simulink model "DvrSimKeybdGD_cs_old"  (R2016a)
settings: Solver=ode5  SolverMode=SingleTasking  StartTime=0.0  StopTime=inf  FixedStep=1/1000  RelTol=1e-3
PreLoadFcn:
  | mbxruntime.callbacks.PreLoadFcn(bdroot);
PostLoadFcn:
  | mbxruntime.callbacks.PostLoadFcn(bdroot);
InitFcn:
  | mbxruntime.callbacks.InitFcn(bdroot);
StartFcn:
  | mbxruntime.callbacks.StartFcn(bdroot);
StopFcn:
  | mbxruntime.callbacks.StopFcn(bdroot);
model workspace (MAT data in the model file):
  mbox_table : struct (value not decoded)
  model_closed = 0
  sim_status = 0
undefined symbols (not defined in the file or in its folder): BMotor1, BMotor2, BrkDelayTime, DControlB, Delay1, Delay2, DiscIntNeverNeededParam, IControlB, JMotor1, JMotor2, PControlB, PreScanCarSimLoadFcn, ratioGearF, ratioGearR, TorqDelayTime, Tstep
undefined symbols (not defined in the file): SteeringColumn, SteeringWheel, WheelL0, WheelL1, WheelR0, WheelR1
libraries: PreScanSimulinkLibrary x35, simulink_extras x26, simulink x26, MyLib x3, Solver_SF x2, pil_lib x1, PreScanUsefulBlocks x1
(part 5 of 12)

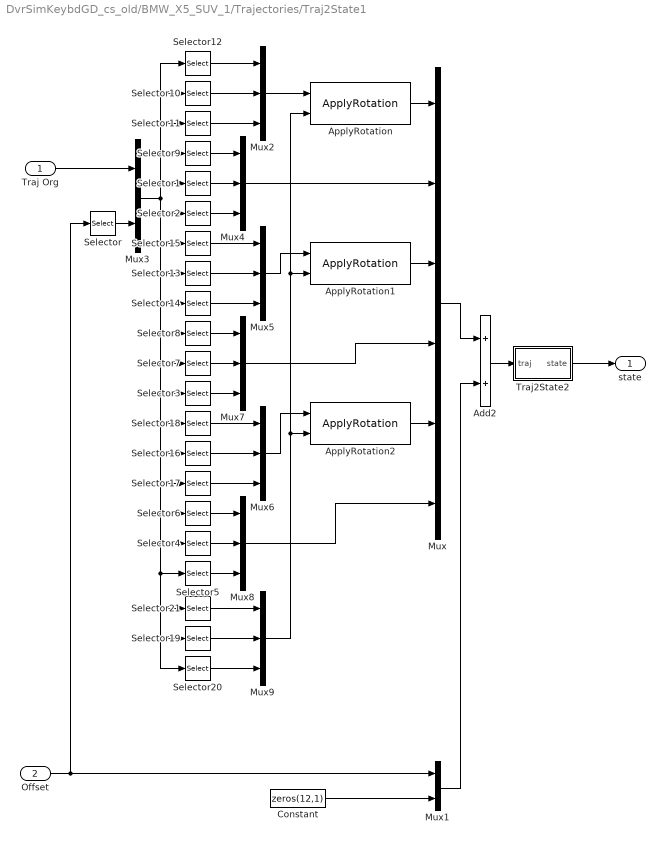
== system DvrSimKeybdGD_cs_old/BMW_X5_SUV_1/Trajectories/Traj2State1 ==
  Traj Org : Inport
  Offset : Inport  Port=2
  Add2 : Sum
  ApplyRotation : PreScanSimulinkLibrary/ApplyRotation
  ApplyRotation1 : PreScanSimulinkLibrary/ApplyRotation
  ApplyRotation2 : PreScanSimulinkLibrary/ApplyRotation
  Constant : Constant  Value=zeros(12,1)
  Mux : Mux  Inputs=6
  Mux1 : Mux  Inputs=2
  Mux{2,4..9} (7 alike) : Mux  Inputs=3
  Mux3 : Mux  Inputs=2
  Selector : Selector  InputPortWidth=6  IndexOptions=Index vector (dialog)  Indices=[4 5 6]  OutputSizes=1
  Selector1 : Selector  InputPortWidth=21  IndexOptions=Index vector (dialog)  Indices=[5]  OutputSizes=1
  Selector10 : Selector  InputPortWidth=21  IndexOptions=Index vector (dialog)  Indices=[2]  OutputSizes=1
  Selector11 : Selector  InputPortWidth=21  IndexOptions=Index vector (dialog)  Indices=[3]  OutputSizes=1
  Selector12 : Selector  InputPortWidth=21  IndexOptions=Index vector (dialog)  Indices=[1]  OutputSizes=1
  Selector13 : Selector  InputPortWidth=21  IndexOptions=Index vector (dialog)  Indices=[8]  OutputSizes=1
  Selector14 : Selector  InputPortWidth=21  IndexOptions=Index vector (dialog)  Indices=[9]  OutputSizes=1
  Selector15 : Selector  InputPortWidth=21  IndexOptions=Index vector (dialog)  Indices=[7]  OutputSizes=1
  Selector16 : Selector  InputPortWidth=21  IndexOptions=Index vector (dialog)  Indices=[14]  OutputSizes=1
  Selector17 : Selector  InputPortWidth=21  IndexOptions=Index vector (dialog)  Indices=[15]  OutputSizes=1
  Selector18 : Selector  InputPortWidth=21  IndexOptions=Index vector (dialog)  Indices=[13]  OutputSizes=1
  Selector19 : Selector  InputPortWidth=21  IndexOptions=Index vector (dialog)  Indices=[20]  OutputSizes=1
  Selector2 : Selector  InputPortWidth=21  IndexOptions=Index vector (dialog)  Indices=[6]  OutputSizes=1
  Selector20 : Selector  InputPortWidth=21  IndexOptions=Index vector (dialog)  Indices=[21]  OutputSizes=1
  Selector21 : Selector  InputPortWidth=21  IndexOptions=Index vector (dialog)  Indices=[19]  OutputSizes=1
  Selector3 : Selector  InputPortWidth=21  IndexOptions=Index vector (dialog)  Indices=[12]  OutputSizes=1
  Selector4 : Selector  InputPortWidth=21  IndexOptions=Index vector (dialog)  Indices=[17]  OutputSizes=1
  Selector5 : Selector  InputPortWidth=21  IndexOptions=Index vector (dialog)  Indices=[18]  OutputSizes=1
  Selector6 : Selector  InputPortWidth=21  IndexOptions=Index vector (dialog)  Indices=[16]  OutputSizes=1
  Selector7 : Selector  InputPortWidth=21  IndexOptions=Index vector (dialog)  Indices=[11]  OutputSizes=1
  Selector8 : Selector  InputPortWidth=21  IndexOptions=Index vector (dialog)  Indices=[10]  OutputSizes=1
  Selector9 : Selector  InputPortWidth=21  IndexOptions=Index vector (dialog)  Indices=[4]  OutputSizes=1
  Traj2State2 : Subsystem
  state : Outport
  wires:
  Mux9/1 -> ApplyRotation2/2, ApplyRotation1/2, ApplyRotation/2
  Selector20/1 -> Mux9/3
  Selector19/1 -> Mux9/2
  Selector21/1 -> Mux9/1
  Selector5/1 -> Mux8/3
  Selector4/1 -> Mux8/2
  Selector6/1 -> Mux8/1
  Mux8/1 -> Mux/6
  Mux6/1 -> ApplyRotation2/1
  Mux7/1 -> Mux/4
  ApplyRotation2/1 -> Mux/5
  Selector3/1 -> Mux7/3
  Selector7/1 -> Mux7/2
  Selector8/1 -> Mux7/1
  Mux4/1 -> Mux/2
  Mux5/1 -> ApplyRotation1/1
  ApplyRotation1/1 -> Mux/3
  Mux2/1 -> ApplyRotation/1
  ApplyRotation/1 -> Mux/1
  Selector2/1 -> Mux4/3
  Selector1/1 -> Mux4/2
  Selector9/1 -> Mux4/1
  Selector17/1 -> Mux6/3
  Selector16/1 -> Mux6/2
  Selector18/1 -> Mux6/1
  Selector14/1 -> Mux5/3
  Selector13/1 -> Mux5/2
  Selector15/1 -> Mux5/1
  Selector11/1 -> Mux2/3
  Selector10/1 -> Mux2/2
  Selector12/1 -> Mux2/1
  Mux3/1 -> Selector8/1, Selector7/1, Selector3/1, Selector18/1, Selector16/1, Selector17/1, Selector6/1, Selector20/1, Selector19/1, Selector21/1, Selector5/1, Selector4/1, Selector14/1, Selector13/1, Selector15/1, Selector2/1, Selector1/1, Selector9/1, Selector12/1, Selector10/1, Selector11/1
  Mux1/1 -> Add2/2
  Constant/1 -> Mux1/2
  Add2/1 -> Traj2State2/1(traj)
  Selector/1 -> Mux3/2
  Traj Org/1 -> Mux3/1
  Offset/1 -> Mux1/1, Selector/1
  Mux/1 -> Add2/1
  Traj2State2/1(state) -> state/1

== system DvrSimKeybdGD_cs_old/BMW_X5_SUV_1/Trajectories/TrajCoGOffset ==
  State In : Inport
  Add : Sum  Inputs=+-+
  Add1 : Sum
  ApplyRotation : PreScanSimulinkLibrary/ApplyRotation
  ApplyRotation1 : PreScanSimulinkLibrary/ApplyRotation
  CoG Offset : Constant  Value=[0 0 CoGOffsetZ]
  Degrees to Radians : simulink_extras/Transformations/Degrees to Radians
  Demux1 : Demux  Outputs=[3 3 3]
  Mux : Mux  Inputs=[3 3 3]
  Orientation : Constant  Value=[InitRoll InitPitch 0]
  State Out : Outport
  wires:
  State In/1 -> Demux1/1
  Demux1/1 -> Add/1
  Add/1 -> Mux/1
  Demux1/3 -> Mux/3, Add1/2
  Mux/1 -> State Out/1
  Demux1/2 -> Mux/2
  Orientation/1 -> Degrees to Radians/1
  ApplyRotation/1 -> Add/3
  ApplyRotation1/1 -> Add/2
  Add1/1 -> ApplyRotation/2
  CoG Offset/1 -> ApplyRotation1/1, ApplyRotation/1
  Degrees to Radians/1 -> Add1/1, ApplyRotation1/2

== system DvrSimKeybdGD_cs_old/BMW_X5_SUV_1/Trajectories/Trajectory_4 ==
  From Workspace : FromWorkspace  VariableName=trajectory  SampleTime=TimeStep  OutputAfterFinalValue=Holding final value
  From Workspace1 : FromWorkspace  VariableName=trajectory  SampleTime=TimeStep  OutputAfterFinalValue=Setting to zero
  Mux : Mux  Inputs=2
  Selector1 : Selector  InputPortWidth=24  IndexOptions=Index vector (dialog)  Indices=[7:18]  OutputSizes=1
  Selector9 : Selector  InputPortWidth=24  IndexOptions=Index vector (dialog)  Indices=[1:6]  OutputSizes=1
  trajectory : Outport
  wires:
  From Workspace/1 -> Selector9/1
  From Workspace1/1 -> Selector1/1
  Mux/1 -> trajectory/1
  Selector9/1 -> Mux/1
  Selector1/1 -> Mux/2

== system DvrSimKeybdGD_cs_old/BMW_Z3_Convertible_1/SELF_Demux/compas converter ==
  rotz [rad] : Inport
  cart2compas : Subsystem
  rad2deg : Gain  Gain=180/pi
  heading [deg] : Outport
  wires:
  rad2deg/1 -> cart2compas/1(Angle [deg])
  rotz [rad]/1 -> rad2deg/1
  cart2compas/1(heading [deg]) -> heading [deg]/1

== system DvrSimKeybdGD_cs_old/BMW_Z3_Convertible_1/Trajectories/ElapsedTrack1 ==
  Offset : Inport
  s : Inport  Port=2
  ApplyRotation : PreScanSimulinkLibrary/ApplyRotation
  Degrees to Radians : simulink_extras/Transformations/Degrees to Radians
  Mux2 : Mux  Inputs=3
  Mux3 : Mux  Inputs=3
  MuxState : Subsystem
  OffsetCor : Subsystem
  Orientation : Constant  Value=[InitRoll InitPitch 0]
  pitchAngle : Lookup  InputValues=s  Table=pitch  LookUpMeth=Interpolation-Use End Values
  rollAngle : Lookup  InputValues=s  Table=roll  LookUpMeth=Interpolation-Use End Values
  xpos : Lookup  InputValues=s  Table=x  LookUpMeth=Interpolation-Use End Values
  yawAngle : Lookup  InputValues=s  Table=yaw  LookUpMeth=Interpolation-Use End Values
  ypos : Lookup  InputValues=s  Table=y  LookUpMeth=Interpolation-Use End Values
  zpos : Lookup  InputValues=s  Table=z  LookUpMeth=Interpolation-Use End Values
  state : Outport
  wires:
  OffsetCor/2(orientation_cor) -> MuxState/2(RPYAngle_[rad])
  OffsetCor/1(pos_cor) -> MuxState/1(xyzPos_[m])
  Mux3/1 -> OffsetCor/2(orientation)
  ApplyRotation/1 -> OffsetCor/1(position)
  yawAngle/1 -> Mux3/3
  pitchAngle/1 -> Mux3/2
  rollAngle/1 -> Mux3/1
  Degrees to Radians/1 -> ApplyRotation/2
  Mux2/1 -> ApplyRotation/1
  Orientation/1 -> Degrees to Radians/1
  zpos/1 -> Mux2/3
  ypos/1 -> Mux2/2
  xpos/1 -> Mux2/1
  MuxState/1(State) -> state/1
  s/1 -> pitchAngle/1, yawAngle/1, rollAngle/1, zpos/1, ypos/1, xpos/1
  Offset/1 -> OffsetCor/3(Offset)

== system DvrSimKeybdGD_cs_old/BMW_Z3_Convertible_1/Trajectories/End of Track is reached ==
  s : Inport
  Relational Operator : RelationalOperator  OutDataTypeStr=boolean
  elapsed distance at end of track : Constant  Value=s(end)
  end_reached : Outport
  wires:
  Relational Operator/1 -> end_reached/1
  s/1 -> Relational Operator/1
  elapsed distance at end of track/1 -> Relational Operator/2

== system DvrSimKeybdGD_cs_old/BMW_Z3_Convertible_1/Trajectories/Traj2State1 ==
  Traj Org : Inport
  Offset : Inport  Port=2
  Add2 : Sum
  ApplyRotation : PreScanSimulinkLibrary/ApplyRotation
  ApplyRotation1 : PreScanSimulinkLibrary/ApplyRotation
  ApplyRotation2 : PreScanSimulinkLibrary/ApplyRotation
  Constant : Constant  Value=zeros(12,1)
  Mux : Mux  Inputs=6
  Mux1 : Mux  Inputs=2
  Mux{2,4..9} (7 alike) : Mux  Inputs=3
  Mux3 : Mux  Inputs=2
  Selector : Selector  InputPortWidth=6  IndexOptions=Index vector (dialog)  Indices=[4 5 6]  OutputSizes=1
  Selector1 : Selector  InputPortWidth=21  IndexOptions=Index vector (dialog)  Indices=[5]  OutputSizes=1
  Selector10 : Selector  InputPortWidth=21  IndexOptions=Index vector (dialog)  Indices=[2]  OutputSizes=1
  Selector11 : Selector  InputPortWidth=21  IndexOptions=Index vector (dialog)  Indices=[3]  OutputSizes=1
  Selector12 : Selector  InputPortWidth=21  IndexOptions=Index vector (dialog)  Indices=[1]  OutputSizes=1
  Selector13 : Selector  InputPortWidth=21  IndexOptions=Index vector (dialog)  Indices=[8]  OutputSizes=1
  Selector14 : Selector  InputPortWidth=21  IndexOptions=Index vector (dialog)  Indices=[9]  OutputSizes=1
  Selector15 : Selector  InputPortWidth=21  IndexOptions=Index vector (dialog)  Indices=[7]  OutputSizes=1
  Selector16 : Selector  InputPortWidth=21  IndexOptions=Index vector (dialog)  Indices=[14]  OutputSizes=1
  Selector17 : Selector  InputPortWidth=21  IndexOptions=Index vector (dialog)  Indices=[15]  OutputSizes=1
  Selector18 : Selector  InputPortWidth=21  IndexOptions=Index vector (dialog)  Indices=[13]  OutputSizes=1
  Selector19 : Selector  InputPortWidth=21  IndexOptions=Index vector (dialog)  Indices=[20]  OutputSizes=1
  Selector2 : Selector  InputPortWidth=21  IndexOptions=Index vector (dialog)  Indices=[6]  OutputSizes=1
  Selector20 : Selector  InputPortWidth=21  IndexOptions=Index vector (dialog)  Indices=[21]  OutputSizes=1
  Selector21 : Selector  InputPortWidth=21  IndexOptions=Index vector (dialog)  Indices=[19]  OutputSizes=1
  Selector3 : Selector  InputPortWidth=21  IndexOptions=Index vector (dialog)  Indices=[12]  OutputSizes=1
  Selector4 : Selector  InputPortWidth=21  IndexOptions=Index vector (dialog)  Indices=[17]  OutputSizes=1
  Selector5 : Selector  InputPortWidth=21  IndexOptions=Index vector (dialog)  Indices=[18]  OutputSizes=1
  Selector6 : Selector  InputPortWidth=21  IndexOptions=Index vector (dialog)  Indices=[16]  OutputSizes=1
  Selector7 : Selector  InputPortWidth=21  IndexOptions=Index vector (dialog)  Indices=[11]  OutputSizes=1
  Selector8 : Selector  InputPortWidth=21  IndexOptions=Index vector (dialog)  Indices=[10]  OutputSizes=1
  Selector9 : Selector  InputPortWidth=21  IndexOptions=Index vector (dialog)  Indices=[4]  OutputSizes=1
  Traj2State2 : Subsystem
  state : Outport
  wires:
  Mux9/1 -> ApplyRotation2/2, ApplyRotation1/2, ApplyRotation/2
  Selector20/1 -> Mux9/3
  Selector19/1 -> Mux9/2
  Selector21/1 -> Mux9/1
  Selector5/1 -> Mux8/3
  Selector4/1 -> Mux8/2
  Selector6/1 -> Mux8/1
  Mux8/1 -> Mux/6
  Mux6/1 -> ApplyRotation2/1
  Mux7/1 -> Mux/4
  ApplyRotation2/1 -> Mux/5
  Selector3/1 -> Mux7/3
  Selector7/1 -> Mux7/2
  Selector8/1 -> Mux7/1
  Mux4/1 -> Mux/2
  Mux5/1 -> ApplyRotation1/1
  ApplyRotation1/1 -> Mux/3
  Mux2/1 -> ApplyRotation/1
  ApplyRotation/1 -> Mux/1
  Selector2/1 -> Mux4/3
  Selector1/1 -> Mux4/2
  Selector9/1 -> Mux4/1
  Selector17/1 -> Mux6/3
  Selector16/1 -> Mux6/2
  Selector18/1 -> Mux6/1
  Selector14/1 -> Mux5/3
  Selector13/1 -> Mux5/2
  Selector15/1 -> Mux5/1
  Selector11/1 -> Mux2/3
  Selector10/1 -> Mux2/2
  Selector12/1 -> Mux2/1
  Mux3/1 -> Selector8/1, Selector7/1, Selector3/1, Selector18/1, Selector16/1, Selector17/1, Selector6/1, Selector20/1, Selector19/1, Selector21/1, Selector5/1, Selector4/1, Selector14/1, Selector13/1, Selector15/1, Selector2/1, Selector1/1, Selector9/1, Selector12/1, Selector10/1, Selector11/1
  Mux1/1 -> Add2/2
  Constant/1 -> Mux1/2
  Add2/1 -> Traj2State2/1(traj)
  Selector/1 -> Mux3/2
  Traj Org/1 -> Mux3/1
  Offset/1 -> Mux1/1, Selector/1
  Mux/1 -> Add2/1
  Traj2State2/1(state) -> state/1

== system DvrSimKeybdGD_cs_old/BMW_Z3_Convertible_1/Trajectories/TrajCoGOffset ==
  State In : Inport
  Add : Sum  Inputs=+-+
  Add1 : Sum
  ApplyRotation : PreScanSimulinkLibrary/ApplyRotation
  ApplyRotation1 : PreScanSimulinkLibrary/ApplyRotation
  CoG Offset : Constant  Value=[0 0 CoGOffsetZ]
  Degrees to Radians : simulink_extras/Transformations/Degrees to Radians
  Demux1 : Demux  Outputs=[3 3 3]
  Mux : Mux  Inputs=[3 3 3]
  Orientation : Constant  Value=[InitRoll InitPitch 0]
  State Out : Outport
  wires:
  State In/1 -> Demux1/1
  Demux1/1 -> Add/1
  Add/1 -> Mux/1
  Demux1/3 -> Mux/3, Add1/2
  Mux/1 -> State Out/1
  Demux1/2 -> Mux/2
  Orientation/1 -> Degrees to Radians/1
  ApplyRotation/1 -> Add/3
  ApplyRotation1/1 -> Add/2
  Add1/1 -> ApplyRotation/2
  CoG Offset/1 -> ApplyRotation1/1, ApplyRotation/1
  Degrees to Radians/1 -> Add1/1, ApplyRotation1/2

== system DvrSimKeybdGD_cs_old/BMW_Z3_Convertible_1/Trajectories/Trajectory_1 ==
  From Workspace : FromWorkspace  VariableName=trajectory  SampleTime=TimeStep  OutputAfterFinalValue=Holding final value
  From Workspace1 : FromWorkspace  VariableName=trajectory  SampleTime=TimeStep  OutputAfterFinalValue=Setting to zero
  Mux : Mux  Inputs=2
  Selector1 : Selector  InputPortWidth=24  IndexOptions=Index vector (dialog)  Indices=[7:18]  OutputSizes=1
  Selector9 : Selector  InputPortWidth=24  IndexOptions=Index vector (dialog)  Indices=[1:6]  OutputSizes=1
  trajectory : Outport
  wires:
  From Workspace/1 -> Selector9/1
  From Workspace1/1 -> Selector1/1
  Mux/1 -> trajectory/1
  Selector9/1 -> Mux/1
  Selector1/1 -> Mux/2

== system DvrSimKeybdGD_cs_old/Ford_Fiesta_Hatchback_1/SELF_Demux/compas converter ==
  rotz [rad] : Inport
  cart2compas : Subsystem
  rad2deg : Gain  Gain=180/pi
  heading [deg] : Outport
  wires:
  rad2deg/1 -> cart2compas/1(Angle [deg])
  rotz [rad]/1 -> rad2deg/1
  cart2compas/1(heading [deg]) -> heading [deg]/1

== system DvrSimKeybdGD_cs_old/Ford_Fiesta_Hatchback_1/Trajectories/ElapsedTrack1 ==
  Offset : Inport
  s : Inport  Port=2
  ApplyRotation : PreScanSimulinkLibrary/ApplyRotation
  Degrees to Radians : simulink_extras/Transformations/Degrees to Radians
  Mux2 : Mux  Inputs=3
  Mux3 : Mux  Inputs=3
  MuxState : Subsystem
  OffsetCor : Subsystem
  Orientation : Constant  Value=[InitRoll InitPitch 0]
  pitchAngle : Lookup  InputValues=s  Table=pitch  LookUpMeth=Interpolation-Use End Values
  rollAngle : Lookup  InputValues=s  Table=roll  LookUpMeth=Interpolation-Use End Values
  xpos : Lookup  InputValues=s  Table=x  LookUpMeth=Interpolation-Use End Values
  yawAngle : Lookup  InputValues=s  Table=yaw  LookUpMeth=Interpolation-Use End Values
  ypos : Lookup  InputValues=s  Table=y  LookUpMeth=Interpolation-Use End Values
  zpos : Lookup  InputValues=s  Table=z  LookUpMeth=Interpolation-Use End Values
  state : Outport
  wires:
  OffsetCor/2(orientation_cor) -> MuxState/2(RPYAngle_[rad])
  OffsetCor/1(pos_cor) -> MuxState/1(xyzPos_[m])
  Mux3/1 -> OffsetCor/2(orientation)
  ApplyRotation/1 -> OffsetCor/1(position)
  yawAngle/1 -> Mux3/3
  pitchAngle/1 -> Mux3/2
  rollAngle/1 -> Mux3/1
  Degrees to Radians/1 -> ApplyRotation/2
  Mux2/1 -> ApplyRotation/1
  Orientation/1 -> Degrees to Radians/1
  zpos/1 -> Mux2/3
  ypos/1 -> Mux2/2
  xpos/1 -> Mux2/1
  MuxState/1(State) -> state/1
  s/1 -> pitchAngle/1, yawAngle/1, rollAngle/1, zpos/1, ypos/1, xpos/1
  Offset/1 -> OffsetCor/3(Offset)

== system DvrSimKeybdGD_cs_old/Ford_Fiesta_Hatchback_1/Trajectories/End of Track is reached ==
  s : Inport
  Relational Operator : RelationalOperator  OutDataTypeStr=boolean
  elapsed distance at end of track : Constant  Value=s(end)
  end_reached : Outport
  wires:
  Relational Operator/1 -> end_reached/1
  s/1 -> Relational Operator/1
  elapsed distance at end of track/1 -> Relational Operator/2

== system DvrSimKeybdGD_cs_old/Ford_Fiesta_Hatchback_1/Trajectories/Traj2State1 ==
  Traj Org : Inport
  Offset : Inport  Port=2
  Add2 : Sum
  ApplyRotation : PreScanSimulinkLibrary/ApplyRotation
  ApplyRotation1 : PreScanSimulinkLibrary/ApplyRotation
  ApplyRotation2 : PreScanSimulinkLibrary/ApplyRotation
  Constant : Constant  Value=zeros(12,1)
  Mux : Mux  Inputs=6
  Mux1 : Mux  Inputs=2
  Mux{2,4..9} (7 alike) : Mux  Inputs=3
  Mux3 : Mux  Inputs=2
  Selector : Selector  InputPortWidth=6  IndexOptions=Index vector (dialog)  Indices=[4 5 6]  OutputSizes=1
  Selector1 : Selector  InputPortWidth=21  IndexOptions=Index vector (dialog)  Indices=[5]  OutputSizes=1
  Selector10 : Selector  InputPortWidth=21  IndexOptions=Index vector (dialog)  Indices=[2]  OutputSizes=1
  Selector11 : Selector  InputPortWidth=21  IndexOptions=Index vector (dialog)  Indices=[3]  OutputSizes=1
  Selector12 : Selector  InputPortWidth=21  IndexOptions=Index vector (dialog)  Indices=[1]  OutputSizes=1
  Selector13 : Selector  InputPortWidth=21  IndexOptions=Index vector (dialog)  Indices=[8]  OutputSizes=1
  Selector14 : Selector  InputPortWidth=21  IndexOptions=Index vector (dialog)  Indices=[9]  OutputSizes=1
  Selector15 : Selector  InputPortWidth=21  IndexOptions=Index vector (dialog)  Indices=[7]  OutputSizes=1
  Selector16 : Selector  InputPortWidth=21  IndexOptions=Index vector (dialog)  Indices=[14]  OutputSizes=1
  Selector17 : Selector  InputPortWidth=21  IndexOptions=Index vector (dialog)  Indices=[15]  OutputSizes=1
  Selector18 : Selector  InputPortWidth=21  IndexOptions=Index vector (dialog)  Indices=[13]  OutputSizes=1
  Selector19 : Selector  InputPortWidth=21  IndexOptions=Index vector (dialog)  Indices=[20]  OutputSizes=1
  Selector2 : Selector  InputPortWidth=21  IndexOptions=Index vector (dialog)  Indices=[6]  OutputSizes=1
  Selector20 : Selector  InputPortWidth=21  IndexOptions=Index vector (dialog)  Indices=[21]  OutputSizes=1
  Selector21 : Selector  InputPortWidth=21  IndexOptions=Index vector (dialog)  Indices=[19]  OutputSizes=1
  Selector3 : Selector  InputPortWidth=21  IndexOptions=Index vector (dialog)  Indices=[12]  OutputSizes=1
  Selector4 : Selector  InputPortWidth=21  IndexOptions=Index vector (dialog)  Indices=[17]  OutputSizes=1
  Selector5 : Selector  InputPortWidth=21  IndexOptions=Index vector (dialog)  Indices=[18]  OutputSizes=1
  Selector6 : Selector  InputPortWidth=21  IndexOptions=Index vector (dialog)  Indices=[16]  OutputSizes=1
  Selector7 : Selector  InputPortWidth=21  IndexOptions=Index vector (dialog)  Indices=[11]  OutputSizes=1
  Selector8 : Selector  InputPortWidth=21  IndexOptions=Index vector (dialog)  Indices=[10]  OutputSizes=1
  Selector9 : Selector  InputPortWidth=21  IndexOptions=Index vector (dialog)  Indices=[4]  OutputSizes=1
  Traj2State2 : Subsystem
  state : Outport
  wires:
  Mux9/1 -> ApplyRotation2/2, ApplyRotation1/2, ApplyRotation/2
  Selector20/1 -> Mux9/3
  Selector19/1 -> Mux9/2
  Selector21/1 -> Mux9/1
  Selector5/1 -> Mux8/3
  Selector4/1 -> Mux8/2
  Selector6/1 -> Mux8/1
  Mux8/1 -> Mux/6
  Mux6/1 -> ApplyRotation2/1
  Mux7/1 -> Mux/4
  ApplyRotation2/1 -> Mux/5
  Selector3/1 -> Mux7/3
  Selector7/1 -> Mux7/2
  Selector8/1 -> Mux7/1
  Mux4/1 -> Mux/2
  Mux5/1 -> ApplyRotation1/1
  ApplyRotation1/1 -> Mux/3
  Mux2/1 -> ApplyRotation/1
  ApplyRotation/1 -> Mux/1
  Selector2/1 -> Mux4/3
  Selector1/1 -> Mux4/2
  Selector9/1 -> Mux4/1
  Selector17/1 -> Mux6/3
  Selector16/1 -> Mux6/2
  Selector18/1 -> Mux6/1
  Selector14/1 -> Mux5/3
  Selector13/1 -> Mux5/2
  Selector15/1 -> Mux5/1
  Selector11/1 -> Mux2/3
  Selector10/1 -> Mux2/2
  Selector12/1 -> Mux2/1
  Mux3/1 -> Selector8/1, Selector7/1, Selector3/1, Selector18/1, Selector16/1, Selector17/1, Selector6/1, Selector20/1, Selector19/1, Selector21/1, Selector5/1, Selector4/1, Selector14/1, Selector13/1, Selector15/1, Selector2/1, Selector1/1, Selector9/1, Selector12/1, Selector10/1, Selector11/1
  Mux1/1 -> Add2/2
  Constant/1 -> Mux1/2
  Add2/1 -> Traj2State2/1(traj)
  Selector/1 -> Mux3/2
  Traj Org/1 -> Mux3/1
  Offset/1 -> Mux1/1, Selector/1
  Mux/1 -> Add2/1
  Traj2State2/1(state) -> state/1

== system DvrSimKeybdGD_cs_old/Ford_Fiesta_Hatchback_1/Trajectories/TrajCoGOffset ==
  State In : Inport
  Add : Sum  Inputs=+-+
  Add1 : Sum
  ApplyRotation : PreScanSimulinkLibrary/ApplyRotation
  ApplyRotation1 : PreScanSimulinkLibrary/ApplyRotation
  CoG Offset : Constant  Value=[0 0 CoGOffsetZ]
  Degrees to Radians : simulink_extras/Transformations/Degrees to Radians
  Demux1 : Demux  Outputs=[3 3 3]
  Mux : Mux  Inputs=[3 3 3]
  Orientation : Constant  Value=[InitRoll InitPitch 0]
  State Out : Outport
  wires:
  State In/1 -> Demux1/1
  Demux1/1 -> Add/1
  Add/1 -> Mux/1
  Demux1/3 -> Mux/3, Add1/2
  Mux/1 -> State Out/1
  Demux1/2 -> Mux/2
  Orientation/1 -> Degrees to Radians/1
  ApplyRotation/1 -> Add/3
  ApplyRotation1/1 -> Add/2
  Add1/1 -> ApplyRotation/2
  CoG Offset/1 -> ApplyRotation1/1, ApplyRotation/1
  Degrees to Radians/1 -> Add1/1, ApplyRotation1/2

== system DvrSimKeybdGD_cs_old/Ford_Fiesta_Hatchback_1/Trajectories/Trajectory_3 ==
  From Workspace : FromWorkspace  VariableName=trajectory  SampleTime=TimeStep  OutputAfterFinalValue=Holding final value
  From Workspace1 : FromWorkspace  VariableName=trajectory  SampleTime=TimeStep  OutputAfterFinalValue=Setting to zero
  Mux : Mux  Inputs=2
  Selector1 : Selector  InputPortWidth=24  IndexOptions=Index vector (dialog)  Indices=[7:18]  OutputSizes=1
  Selector9 : Selector  InputPortWidth=24  IndexOptions=Index vector (dialog)  Indices=[1:6]  OutputSizes=1
  trajectory : Outport
  wires:
  From Workspace/1 -> Selector9/1
  From Workspace1/1 -> Selector1/1
  Mux/1 -> trajectory/1
  Selector9/1 -> Mux/1
  Selector1/1 -> Mux/2

== system DvrSimKeybdGD_cs_old/Roewe_550_S_Sedan_1/AIR_1_Demux/Activate_Switch ==
  BeamID : Inport
  Heading : Inport  Port=2
  Constant : Constant  Value=0
  Product1 : Product  RndMeth=Zero
  Relational Operator : RelationalOperator  Operator=~=  OutDataTypeStr=boolean
  On/Off : Outport
  wires:
  Constant/1 -> Relational Operator/1
  Relational Operator/1 -> Product1/1
  BeamID/1 -> Relational Operator/2
  Product1/1 -> On/Off/1
  Heading/1 -> Product1/2

== system DvrSimKeybdGD_cs_old/Roewe_550_S_Sedan_1/AIR_1_Demux/Signal2ArrayOfSignals1 ==
  note: Set mask parameter VECTORLENGTH
      |  to MAXMESSAGES
  note: Initial state of Previous vector block
      | set to zeros(VECTORLENGTH,1)
  LoopIndex : Inport
  Element : Inport  Port=2
  Assignment : Assignment  IndexOptions=Index vector (port)  Indices=1  OutputSizes=1
  Previous vector : Memory  X0=zeros(VECTORLENGTH,1)  InheritSampleTime=on
  ArrayofElements : Outport
  wires:
  Element/1 -> Assignment/2
  LoopIndex/1 -> Assignment/3
  Previous vector/1 -> Assignment/1
  Assignment/1 -> ArrayofElements/1, Previous vector/1

== system DvrSimKeybdGD_cs_old/Roewe_550_S_Sedan_1/AIR_1_Demux/Signal2ArrayOfSignals2 ==
  note: Set mask parameter VECTORLENGTH
      |  to MAXMESSAGES
  note: Initial state of Previous vector block
      | set to zeros(VECTORLENGTH,1)
  LoopIndex : Inport
  Element : Inport  Port=2
  Assignment : Assignment  IndexOptions=Index vector (port)  Indices=1  OutputSizes=1
  Previous vector : Memory  X0=zeros(VECTORLENGTH,1)  InheritSampleTime=on
  ArrayofElements : Outport
  wires:
  Element/1 -> Assignment/2
  LoopIndex/1 -> Assignment/3
  Previous vector/1 -> Assignment/1
  Assignment/1 -> ArrayofElements/1, Previous vector/1

== system DvrSimKeybdGD_cs_old/Roewe_550_S_Sedan_1/AIR_1_Demux/Signal2ArrayOfSignals3 ==
  note: Set mask parameter VECTORLENGTH
      |  to MAXMESSAGES
  note: Initial state of Previous vector block
      | set to zeros(VECTORLENGTH,1)
  LoopIndex : Inport
  Element : Inport  Port=2
  Assignment : Assignment  IndexOptions=Index vector (port)  Indices=1  OutputSizes=1
  Previous vector : Memory  X0=zeros(VECTORLENGTH,1)  InheritSampleTime=on
  ArrayofElements : Outport
  wires:
  Element/1 -> Assignment/2
  LoopIndex/1 -> Assignment/3
  Previous vector/1 -> Assignment/1
  Assignment/1 -> ArrayofElements/1, Previous vector/1

== system DvrSimKeybdGD_cs_old/Roewe_550_S_Sedan_1/AIR_1_Demux/Signal2ArrayOfSignals4 ==
  note: Set mask parameter VECTORLENGTH
      |  to MAXMESSAGES
  note: Initial state of Previous vector block
      | set to zeros(VECTORLENGTH,1)
  LoopIndex : Inport
  Element : Inport  Port=2
  Assignment : Assignment  IndexOptions=Index vector (port)  Indices=1  OutputSizes=1
  Previous vector : Memory  X0=zeros(VECTORLENGTH,1)  InheritSampleTime=on
  ArrayofElements : Outport
  wires:
  Element/1 -> Assignment/2
  LoopIndex/1 -> Assignment/3
  Previous vector/1 -> Assignment/1
  Assignment/1 -> ArrayofElements/1, Previous vector/1

== system DvrSimKeybdGD_cs_old/Roewe_550_S_Sedan_1/AIR_1_Demux/Signal2ArrayOfSignals5 ==
  note: Set mask parameter VECTORLENGTH
      |  to MAXMESSAGES
  note: Initial state of Previous vector block
      | set to zeros(VECTORLENGTH,1)
  LoopIndex : Inport
  Element : Inport  Port=2
  Assignment : Assignment  IndexOptions=Index vector (port)  Indices=1  OutputSizes=1
  Previous vector : Memory  X0=zeros(VECTORLENGTH,1)  InheritSampleTime=on
  ArrayofElements : Outport
  wires:
  Element/1 -> Assignment/2
  LoopIndex/1 -> Assignment/3
  Previous vector/1 -> Assignment/1
  Assignment/1 -> ArrayofElements/1, Previous vector/1

== system DvrSimKeybdGD_cs_old/Roewe_550_S_Sedan_1/AIR_1_Demux/Signal2ArrayOfSignals6 ==
  note: Set mask parameter VECTORLENGTH
      |  to MAXMESSAGES
  note: Initial state of Previous vector block
      | set to zeros(VECTORLENGTH,1)
  LoopIndex : Inport
  Element : Inport  Port=2
  Assignment : Assignment  IndexOptions=Index vector (port)  Indices=1  OutputSizes=1
  Previous vector : Memory  X0=zeros(VECTORLENGTH,1)  InheritSampleTime=on
  ArrayofElements : Outport
  wires:
  Element/1 -> Assignment/2
  LoopIndex/1 -> Assignment/3
  Previous vector/1 -> Assignment/1
  Assignment/1 -> ArrayofElements/1, Previous vector/1

== system DvrSimKeybdGD_cs_old/Roewe_550_S_Sedan_1/CarSim I//O/ACCAEB ==
  ACCAEBIn : Inport  OutDataTypeStr=Bus: AccAebInputs  BusOutputAsStruct=on
  ACCAEB_sfcn : pil_lib/PIL Block  SimulationMode=SIL  IsTopModelPIL=off  CodeDir=D:\Temp\SimCodeGen\Dest\ACCAEB_ert_rtw  ConfigName=Software-in-the-Loop (SIL)
  __InputSSForSFun__ : Subsystem
  __OutputSSForSFun__ : Subsystem
  ACCAEBOut : Outport
  wires:
  ACCAEBIn/1 -> __InputSSForSFun__/1(ACCAEBIn)
  __InputSSForSFun__/1(__UniqueOutportName__1__) -> ACCAEB_sfcn/1
  ACCAEB_sfcn/1 -> __OutputSSForSFun__/1(__UniqueInportName__1__)
  ACCAEB_sfcn/2 -> __OutputSSForSFun__/2(__UniqueInportName__2__)
  ACCAEB_sfcn/3 -> __OutputSSForSFun__/3(__UniqueInportName__3__)
  ACCAEB_sfcn/4 -> __OutputSSForSFun__/4(__UniqueInportName__4__)
  ACCAEB_sfcn/5 -> __OutputSSForSFun__/5(__UniqueInportName__5__)
  ACCAEB_sfcn/6 -> __OutputSSForSFun__/6(__UniqueInportName__6__)
  ACCAEB_sfcn/7 -> __OutputSSForSFun__/7(__UniqueInportName__7__)
  ACCAEB_sfcn/8 -> __OutputSSForSFun__/8(__UniqueInportName__8__)
  ACCAEB_sfcn/9 -> __OutputSSForSFun__/9(__UniqueInportName__9__)
  ACCAEB_sfcn/10 -> __OutputSSForSFun__/10(__UniqueInportName__10__)
  ACCAEB_sfcn/11 -> __OutputSSForSFun__/11(__UniqueInportName__11__)
  ACCAEB_sfcn/12 -> __OutputSSForSFun__/12(__UniqueInportName__12__)
  ACCAEB_sfcn/13 -> __OutputSSForSFun__/13(__UniqueInportName__13__)
  ACCAEB_sfcn/14 -> __OutputSSForSFun__/14(__UniqueInportName__14__)
  ACCAEB_sfcn/15 -> __OutputSSForSFun__/15(__UniqueInportName__15__)
  ACCAEB_sfcn/16 -> __OutputSSForSFun__/16(__UniqueInportName__16__)
  ACCAEB_sfcn/17 -> __OutputSSForSFun__/17(__UniqueInportName__17__)
  ACCAEB_sfcn/18 -> __OutputSSForSFun__/18(__UniqueInportName__18__)
  ACCAEB_sfcn/19 -> __OutputSSForSFun__/19(__UniqueInportName__19__)
  ACCAEB_sfcn/20 -> __OutputSSForSFun__/20(__UniqueInportName__20__)
  ACCAEB_sfcn/21 -> __OutputSSForSFun__/21(__UniqueInportName__21__)
  ACCAEB_sfcn/22 -> __OutputSSForSFun__/22(__UniqueInportName__22__)
  ACCAEB_sfcn/23 -> __OutputSSForSFun__/23(__UniqueInportName__23__)
  ACCAEB_sfcn/24 -> __OutputSSForSFun__/24(__UniqueInportName__24__)
  ACCAEB_sfcn/25 -> __OutputSSForSFun__/25(__UniqueInportName__25__)
  ACCAEB_sfcn/26 -> __OutputSSForSFun__/26(__UniqueInportName__26__)
  ACCAEB_sfcn/27 -> __OutputSSForSFun__/27(__UniqueInportName__27__)
  ACCAEB_sfcn/28 -> __OutputSSForSFun__/28(__UniqueInportName__28__)
  ACCAEB_sfcn/29 -> __OutputSSForSFun__/29(__UniqueInportName__29__)
  ACCAEB_sfcn/30 -> __OutputSSForSFun__/30(__UniqueInportName__30__)
  ACCAEB_sfcn/31 -> __OutputSSForSFun__/31(__UniqueInportName__31__)
  ACCAEB_sfcn/32 -> __OutputSSForSFun__/32(__UniqueInportName__32__)
  ACCAEB_sfcn/33 -> __OutputSSForSFun__/33(__UniqueInportName__33__)
  ACCAEB_sfcn/34 -> __OutputSSForSFun__/34(__UniqueInportName__34__)
  ACCAEB_sfcn/35 -> __OutputSSForSFun__/35(__UniqueInportName__35__)
  ACCAEB_sfcn/36 -> __OutputSSForSFun__/36(__UniqueInportName__36__)
  ACCAEB_sfcn/37 -> __OutputSSForSFun__/37(__UniqueInportName__37__)
  ACCAEB_sfcn/38 -> __OutputSSForSFun__/38(__UniqueInportName__38__)
  ACCAEB_sfcn/39 -> __OutputSSForSFun__/39(__UniqueInportName__39__)
  ACCAEB_sfcn/40 -> __OutputSSForSFun__/40(__UniqueInportName__40__)
  ACCAEB_sfcn/41 -> __OutputSSForSFun__/41(__UniqueInportName__41__)
  ACCAEB_sfcn/42 -> __OutputSSForSFun__/42(__UniqueInportName__42__)
  ACCAEB_sfcn/43 -> __OutputSSForSFun__/43(__UniqueInportName__43__)
  ACCAEB_sfcn/44 -> __OutputSSForSFun__/44(__UniqueInportName__44__)
  ACCAEB_sfcn/45 -> __OutputSSForSFun__/45(__UniqueInportName__45__)
  ACCAEB_sfcn/46 -> __OutputSSForSFun__/46(__UniqueInportName__46__)
  ACCAEB_sfcn/47 -> __OutputSSForSFun__/47(__UniqueInportName__47__)
  ACCAEB_sfcn/48 -> __OutputSSForSFun__/48(__UniqueInportName__48__)
  ACCAEB_sfcn/49 -> __OutputSSForSFun__/49(__UniqueInportName__49__)
  ACCAEB_sfcn/50 -> __OutputSSForSFun__/50(__UniqueInportName__50__)
  ACCAEB_sfcn/51 -> __OutputSSForSFun__/51(__UniqueInportName__51__)
  ACCAEB_sfcn/52 -> __OutputSSForSFun__/52(__UniqueInportName__52__)
  ACCAEB_sfcn/53 -> __OutputSSForSFun__/53(__UniqueInportName__53__)
  ACCAEB_sfcn/54 -> __OutputSSForSFun__/54(__UniqueInportName__54__)
  ACCAEB_sfcn/55 -> __OutputSSForSFun__/55(__UniqueInportName__55__)
  ACCAEB_sfcn/56 -> __OutputSSForSFun__/56(__UniqueInportName__56__)
  ACCAEB_sfcn/57 -> __OutputSSForSFun__/57(__UniqueInportName__57__)
  ACCAEB_sfcn/58 -> __OutputSSForSFun__/58(__UniqueInportName__58__)
  ACCAEB_sfcn/59 -> __OutputSSForSFun__/59(__UniqueInportName__59__)
  ACCAEB_sfcn/60 -> __OutputSSForSFun__/60(__UniqueInportName__60__)
  ACCAEB_sfcn/61 -> __OutputSSForSFun__/61(__UniqueInportName__61__)
  ACCAEB_sfcn/62 -> __OutputSSForSFun__/62(__UniqueInportName__62__)
  ACCAEB_sfcn/63 -> __OutputSSForSFun__/63(__UniqueInportName__63__)
  ACCAEB_sfcn/64 -> __OutputSSForSFun__/64(__UniqueInportName__64__)
  ACCAEB_sfcn/65 -> __OutputSSForSFun__/65(__UniqueInportName__65__)
  ACCAEB_sfcn/66 -> __OutputSSForSFun__/66(__UniqueInportName__66__)
  ACCAEB_sfcn/67 -> __OutputSSForSFun__/67(__UniqueInportName__67__)
  ACCAEB_sfcn/68 -> __OutputSSForSFun__/68(__UniqueInportName__68__)
  ACCAEB_sfcn/69 -> __OutputSSForSFun__/69(__UniqueInportName__69__)
  ACCAEB_sfcn/70 -> __OutputSSForSFun__/70(__UniqueInportName__70__)
  ACCAEB_sfcn/71 -> __OutputSSForSFun__/71(__UniqueInportName__71__)
  ACCAEB_sfcn/72 -> __OutputSSForSFun__/72(__UniqueInportName__72__)
  ACCAEB_sfcn/73 -> __OutputSSForSFun__/73(__UniqueInportName__73__)
  ACCAEB_sfcn/74 -> __OutputSSForSFun__/74(__UniqueInportName__74__)
  ACCAEB_sfcn/75 -> __OutputSSForSFun__/75(__UniqueInportName__75__)
  ACCAEB_sfcn/76 -> __OutputSSForSFun__/76(__UniqueInportName__76__)
  ACCAEB_sfcn/77 -> __OutputSSForSFun__/77(__UniqueInportName__77__)
  ACCAEB_sfcn/78 -> __OutputSSForSFun__/78(__UniqueInportName__78__)
  ACCAEB_sfcn/79 -> __OutputSSForSFun__/79(__UniqueInportName__79__)
  ACCAEB_sfcn/80 -> __OutputSSForSFun__/80(__UniqueInportName__80__)
  ACCAEB_sfcn/81 -> __OutputSSForSFun__/81(__UniqueInportName__81__)
  ACCAEB_sfcn/82 -> __OutputSSForSFun__/82(__UniqueInportName__82__)
  ACCAEB_sfcn/83 -> __OutputSSForSFun__/83(__UniqueInportName__83__)
  ACCAEB_sfcn/84 -> __OutputSSForSFun__/84(__UniqueInportName__84__)
  ACCAEB_sfcn/85 -> __OutputSSForSFun__/85(__UniqueInportName__85__)
  ACCAEB_sfcn/86 -> __OutputSSForSFun__/86(__UniqueInportName__86__)
  ACCAEB_sfcn/87 -> __OutputSSForSFun__/87(__UniqueInportName__87__)
  ACCAEB_sfcn/88 -> __OutputSSForSFun__/88(__UniqueInportName__88__)
  ACCAEB_sfcn/89 -> __OutputSSForSFun__/89(__UniqueInportName__89__)
  ACCAEB_sfcn/90 -> __OutputSSForSFun__/90(__UniqueInportName__90__)
  ACCAEB_sfcn/91 -> __OutputSSForSFun__/91(__UniqueInportName__91__)
  ACCAEB_sfcn/92 -> __OutputSSForSFun__/92(__UniqueInportName__92__)
  ACCAEB_sfcn/93 -> __OutputSSForSFun__/93(__UniqueInportName__93__)
  ACCAEB_sfcn/94 -> __OutputSSForSFun__/94(__UniqueInportName__94__)
  ACCAEB_sfcn/95 -> __OutputSSForSFun__/95(__UniqueInportName__95__)
  ACCAEB_sfcn/96 -> __OutputSSForSFun__/96(__UniqueInportName__96__)
  ACCAEB_sfcn/97 -> __OutputSSForSFun__/97(__UniqueInportName__97__)
  ACCAEB_sfcn/98 -> __OutputSSForSFun__/98(__UniqueInportName__98__)
  __OutputSSForSFun__/1(ACCAEBOut) -> ACCAEBOut/1
